simulink model "sla_vip_filter_vector"  (R2015b)
settings: Solver=FixedStepDiscrete  SolverMode=SingleTasking  StartTime=0.0  StopTime=1  RelTol=1e-3
PreLoadFcn:
  | Param_vip_vector
values from neighbouring files (symbols this model uses):
  Hvector = reshape(H, TAP*TAP, 1)    [Param_vip_vector.m]
  TAP = 5    [Param_vip_vector.m]
undefined symbols (not defined in the file or in its folder): LineBuf, TAPDly
libraries: simulink x11, dspobslib x10, visionsinks x3, dspsigattribs x2, dspvision x1, visionfilter x1, dspindex x1
settings Model: Creator=amatsumo  LastModifiedBy=amatsumo
settings DataIOCC: SaveFormat=Array  SignalLoggingSaveFormat=ModelDataLogs  SaveOutput=off  SignalLogging=off  SaveTime=off
settings OptimizationCC: BlockReduction=off  ConditionallyExecuteInputs=off  DefaultParameterBehavior=Inlined  ExpressionDepthLimit=2147483647
settings DebuggingCC: AlgebraicLoopMsg=error  UnderspecifiedInitializationDetection=Classic  MergeDetectMultiDrivingBlocksExec=none  SolverPrmCheckMsg=warning  InheritedTsInSrcMsg=none  SingleTaskRateTransMsg=error  ParameterPrecisionLossMsg=none  FcnCallInpInsideContextMsg=UseLocalSettings  StateNameClashWarn=warning
settings HardwareCC: ProdBitPerPointer=32  ProdLargestAtomicFloat=None  ProdIntDivRoundTo=Undefined  ProdEndianess=Unspecified  ProdWordSize=32  ProdHWDeviceType=ASIC/FPGA->ASIC/FPGA  TargetBitPerPointer=64  TargetLongLongMode=on  TargetIntDivRoundTo=Zero  TargetEndianess=LittleEndian  TargetWordSize=64  TargetHWDeviceType=MATLAB Host  ProdEqTarget=off
settings RTWCC: CustomInclude=C:\altera\12.0\modelsim_ase\include
settings GRTTargetCC: GeneratePreprocessorConditionals=Disable all  CombineOutputUpdateFcns=off  GRTInterface=on
settings ConfigComp: CovModelRefEnable=Off  CovSFcnEnable=off

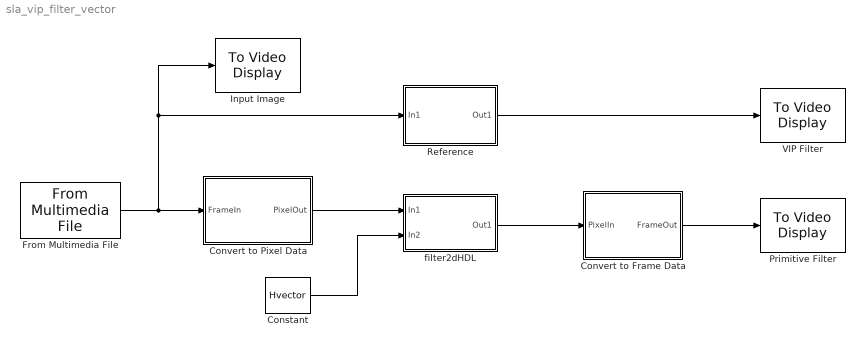
== system sla_vip_filter_vector ==
  Constant : Constant  Value=Hvector  OutDataTypeStr=dt_Hvector  SampleTime=-1
  Convert to Frame Data : Subsystem
  Convert to Pixel Data : Subsystem
  From Multimedia File : dspvision/From Multimedia File  inputFilename=vipmen.avi  loop=on  numPlays=inf  outputStreams=Video only  videoDataType=double  audioDataType=int16  inheritSampleTime=off  userDefinedSampleTime=1/24  noAudioOutput=off  isIntensityVideo=off  fourcc=Intensity  colorVideoFormat=Separate color signals  outputEOF=off  dataOrg=Column-major  audioFrameSize=1024  computeAudioFrameSize=off  outSamplingMode=Frame based
  Input Image : visionsinks/To Video Display  windowSizeMode=True size (1:1)  openAtMdlStart=on  fullScreen=off  videoWindowX=738  videoWindowY=-9  saveWindowSize=off  videoWindowWidth=160  videoWindowHeight=120  inputColorFormat=RGB  inputType=Obsolete  imagePorts=One multidimensional signal  OutputDevice=On-screen video monitor  dataOrg=Column-major  isWindowOpen=on
  Primitive Filter : visionsinks/To Video Display  windowSizeMode=True size (1:1)  openAtMdlStart=on  fullScreen=off  videoWindowX=1083  videoWindowY=-9  saveWindowSize=off  videoWindowWidth=160  videoWindowHeight=120  inputColorFormat=RGB  inputType=Obsolete  imagePorts=One multidimensional signal  OutputDevice=On-screen video monitor  dataOrg=Column-major  isWindowOpen=on
  Reference : Subsystem
  VIP Filter : visionsinks/To Video Display  windowSizeMode=True size (1:1)  openAtMdlStart=on  fullScreen=off  videoWindowX=908  videoWindowY=-9  saveWindowSize=off  videoWindowWidth=160  videoWindowHeight=120  inputColorFormat=RGB  inputType=Obsolete  imagePorts=One multidimensional signal  OutputDevice=On-screen video monitor  dataOrg=Column-major  isWindowOpen=on
  filter2dHDL : Subsystem
  wires:
  From Multimedia File/1 -> Convert to Pixel Data/1(FrameIn), Reference/1(In1), Input Image/1
  Reference/1(Out1) -> VIP Filter/1
  Convert to Frame Data/1(FrameOut) -> Primitive Filter/1
  Convert to Pixel Data/1(PixelOut) -> filter2dHDL/1(In1)
  filter2dHDL/1(Out1) -> Convert to Frame Data/1(PixelIn)
  Constant/1 -> filter2dHDL/2(In2)

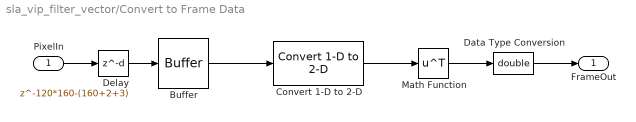
== system sla_vip_filter_vector/Convert to Frame Data ==
  PixelIn : Inport
  Buffer : Buffer  N=160*120  TreatMby1Signals=One channel
  Convert 1-D to 2-D : dspsigattribs/Convert 1-D to 2-D  M=160  N=120  frameBasedOut=off
  Data Type Conversion : DataTypeConversion  OutDataTypeStr=double  SaturateOnIntegerOverflow=on
  Delay : Delay  DelayLength=120*160-(160+2+3)  InitialCondition=0
  Math Function : Math  Operator=transpose  SaturateOnIntegerOverflow=on
  FrameOut : Outport
  wires:
  Buffer/1 -> Convert 1-D to 2-D/1
  Convert 1-D to 2-D/1 -> Math Function/1
  PixelIn/1 -> Delay/1
  Delay/1 -> Buffer/1
  Data Type Conversion/1 -> FrameOut/1
  Math Function/1 -> Data Type Conversion/1

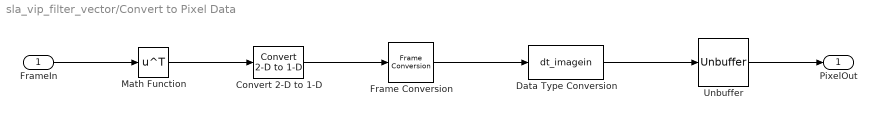
== system sla_vip_filter_vector/Convert to Pixel Data ==
  FrameIn : Inport
  Convert 2-D to 1-D : dspsigattribs/Convert 2-D to 1-D
  Data Type Conversion : DataTypeConversion  OutDataTypeStr=dt_imagein  SaturateOnIntegerOverflow=on
  Frame Conversion : FrameConversion  InheritSamplingMode=off
  Math Function : Math  Operator=transpose  SaturateOnIntegerOverflow=on
  Unbuffer : Unbuffer  SampleBasedProcessing=Same as frame based
  PixelOut : Outport
  wires:
  Frame Conversion/1 -> Data Type Conversion/1
  Convert 2-D to 1-D/1 -> Frame Conversion/1
  FrameIn/1 -> Math Function/1
  Unbuffer/1 -> PixelOut/1
  Data Type Conversion/1 -> Unbuffer/1
  Math Function/1 -> Convert 2-D to 1-D/1

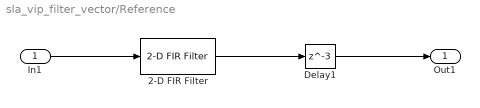
== system sla_vip_filter_vector/Reference ==
  In1 : Inport
  2-D FIR Filter : visionfilter/2-D FIR Filter  separable=off  filtSrc=Specify via dialog  filterMtrx=H  verticalFilter=[4 0]  horizontalFilter=[4 0]  outSize=Same as input port I  padType=Constant  padSrc=Specify via dialog  padVal=0  method=Convolution  firstCoeffMode=Binary point scaling  firstCoeffWordLength=8  firstCoeffFracLength=4  firstCoeffSignedness=Signed  firstCoeffDataTypeStr=fixdt(1,8,4)  firstCoeffLastDataTypeStr=fixdt(1,8,4)  firstCoeffMin=[]  firstCoeffMax=[]  outputMode=Binary point scaling  outputWordLength=20  outputFracLength=4  outputSignedness=Auto  outputDataTypeStr=fixdt([],20,4)  outputLastDataTypeStr=fixdt([],20,4)  outputMin=[]  outputMax=[]  accumDataTypeStr=Inherit: Same as product output  accumLastDataTypeStr=Inherit: Same as product output  prodOutputMode=Binary point scaling  prodOutputWordLength=16  prodOutputFracLength=4  prodOutputDataTypeStr=fixdt([],16,4)  prodOutputLastDataTypeStr=fixdt([],16,4)  roundingMode=Floor  overflowMode=on
  Delay1 : Delay  DelayLength=3  InitialCondition=0
  Out1 : Outport
  wires:
  Delay1/1 -> Out1/1
  2-D FIR Filter/1 -> Delay1/1
  In1/1 -> 2-D FIR Filter/1

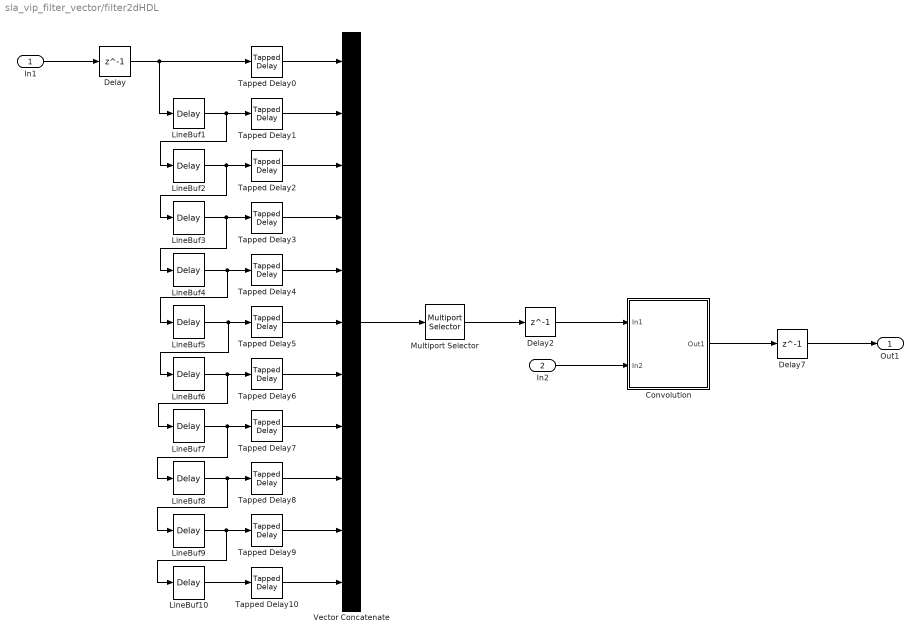
== system sla_vip_filter_vector/filter2dHDL ==
  In1 : Inport
  In2 : Inport  Port=2
  Convolution : Subsystem
  Delay : Delay  DelayLength=1
  Delay2 : Delay  DelayLength=1
  Delay7 : Delay  DelayLength=1
  LineBuf1 : dspobslib/Delay  InputProcessing=Columns as channels (frame based)  dly_unit=Samples  delay=LineBuf(1)  ic_detail=off  dif_ic_for_ch=off  dif_ic_for_dly=off  ic=0  reset_popup=None
  LineBuf10 : dspobslib/Delay  InputProcessing=Columns as channels (frame based)  dly_unit=Samples  delay=LineBuf(10)  ic_detail=off  dif_ic_for_ch=off  dif_ic_for_dly=off  ic=0  reset_popup=None
  LineBuf2 : dspobslib/Delay  InputProcessing=Columns as channels (frame based)  dly_unit=Samples  delay=LineBuf(2)  ic_detail=off  dif_ic_for_ch=off  dif_ic_for_dly=off  ic=0  reset_popup=None
  LineBuf3 : dspobslib/Delay  InputProcessing=Columns as channels (frame based)  dly_unit=Samples  delay=LineBuf(3)  ic_detail=off  dif_ic_for_ch=off  dif_ic_for_dly=off  ic=0  reset_popup=None
  LineBuf4 : dspobslib/Delay  InputProcessing=Columns as channels (frame based)  dly_unit=Samples  delay=LineBuf(4)  ic_detail=off  dif_ic_for_ch=off  dif_ic_for_dly=off  ic=0  reset_popup=None
  LineBuf5 : dspobslib/Delay  InputProcessing=Columns as channels (frame based)  dly_unit=Samples  delay=LineBuf(5)  ic_detail=off  dif_ic_for_ch=off  dif_ic_for_dly=off  ic=0  reset_popup=None
  LineBuf6 : dspobslib/Delay  InputProcessing=Columns as channels (frame based)  dly_unit=Samples  delay=LineBuf(6)  ic_detail=off  dif_ic_for_ch=off  dif_ic_for_dly=off  ic=0  reset_popup=None
  LineBuf7 : dspobslib/Delay  InputProcessing=Columns as channels (frame based)  dly_unit=Samples  delay=LineBuf(7)  ic_detail=off  dif_ic_for_ch=off  dif_ic_for_dly=off  ic=0  reset_popup=None
  LineBuf8 : dspobslib/Delay  InputProcessing=Columns as channels (frame based)  dly_unit=Samples  delay=LineBuf(8)  ic_detail=off  dif_ic_for_ch=off  dif_ic_for_dly=off  ic=0  reset_popup=None
  LineBuf9 : dspobslib/Delay  InputProcessing=Columns as channels (frame based)  dly_unit=Samples  delay=LineBuf(9)  ic_detail=off  dif_ic_for_ch=off  dif_ic_for_dly=off  ic=0  reset_popup=None
  Multiport Selector : dspindex/Multiport Selector  rowsOrCols=Rows  idxCellArray=[ 1: (TAP*TAP) ]  idxErrMode=Clip Index
  Tapped Delay0 : simulink/Discrete/Tapped Delay  vinit=0.0  samptime=-1  NumDelays=TAP  DelayOrder=Newest  includeCurrent=off
  Tapped Delay1 : simulink/Discrete/Tapped Delay  vinit=0.0  samptime=-1  NumDelays=TAPDly(1)  DelayOrder=Newest  includeCurrent=off
  Tapped Delay10 : simulink/Discrete/Tapped Delay  vinit=0.0  samptime=-1  NumDelays=TAPDly(10)  DelayOrder=Newest  includeCurrent=off
  Tapped Delay2 : simulink/Discrete/Tapped Delay  vinit=0.0  samptime=-1  NumDelays=TAPDly(2)  DelayOrder=Newest  includeCurrent=off
  Tapped Delay3 : simulink/Discrete/Tapped Delay  vinit=0.0  samptime=-1  NumDelays=TAPDly(3)  DelayOrder=Newest  includeCurrent=off
  Tapped Delay4 : simulink/Discrete/Tapped Delay  vinit=0.0  samptime=-1  NumDelays=TAPDly(4)  DelayOrder=Newest  includeCurrent=off
  Tapped Delay5 : simulink/Discrete/Tapped Delay  vinit=0.0  samptime=-1  NumDelays=TAPDly(5)  DelayOrder=Newest  includeCurrent=off
  Tapped Delay6 : simulink/Discrete/Tapped Delay  vinit=0.0  samptime=-1  NumDelays=TAPDly(6)  DelayOrder=Newest  includeCurrent=off
  Tapped Delay7 : simulink/Discrete/Tapped Delay  vinit=0.0  samptime=-1  NumDelays=TAPDly(7)  DelayOrder=Newest  includeCurrent=off
  Tapped Delay8 : simulink/Discrete/Tapped Delay  vinit=0.0  samptime=-1  NumDelays=TAPDly(8)  DelayOrder=Newest  includeCurrent=off
  Tapped Delay9 : simulink/Discrete/Tapped Delay  vinit=0.0  samptime=-1  NumDelays=TAPDly(9)  DelayOrder=Newest  includeCurrent=off
  Vector Concatenate : Concatenate  NumInputs=11
  Out1 : Outport
  wires:
  Delay7/1 -> Out1/1
  In1/1 -> Delay/1
  LineBuf1/1 -> LineBuf2/1, Tapped Delay1/1
  Delay/1 -> Tapped Delay0/1, LineBuf1/1
  Tapped Delay1/1 -> Vector Concatenate/2
  LineBuf2/1 -> Tapped Delay2/1, LineBuf3/1
  LineBuf3/1 -> LineBuf4/1, Tapped Delay3/1
  LineBuf4/1 -> LineBuf5/1, Tapped Delay4/1
  Tapped Delay2/1 -> Vector Concatenate/3
  Tapped Delay3/1 -> Vector Concatenate/4
  Tapped Delay4/1 -> Vector Concatenate/5
  Tapped Delay0/1 -> Vector Concatenate/1
  Tapped Delay5/1 -> Vector Concatenate/6
  LineBuf5/1 -> Tapped Delay5/1, LineBuf6/1
  Tapped Delay6/1 -> Vector Concatenate/7
  Vector Concatenate/1 -> Multiport Selector/1
  Tapped Delay7/1 -> Vector Concatenate/8
  LineBuf6/1 -> LineBuf7/1, Tapped Delay6/1
  LineBuf10/1 -> Tapped Delay10/1
  Tapped Delay8/1 -> Vector Concatenate/9
  Tapped Delay9/1 -> Vector Concatenate/10
  Tapped Delay10/1 -> Vector Concatenate/11
  LineBuf7/1 -> LineBuf8/1, Tapped Delay7/1
  LineBuf8/1 -> LineBuf9/1, Tapped Delay8/1
  LineBuf9/1 -> LineBuf10/1, Tapped Delay9/1
  Delay2/1 -> Convolution/1(In1)
  In2/1 -> Convolution/2(In2)
  Convolution/1(Out1) -> Delay7/1
  Multiport Selector/1 -> Delay2/1

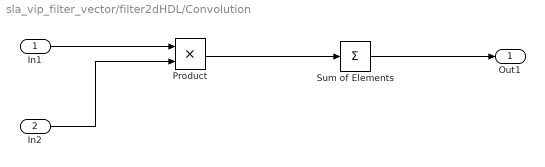
== system sla_vip_filter_vector/filter2dHDL/Convolution ==
  In1 : Inport
  In2 : Inport  Port=2
  Product : Product  OutDataTypeStr=dt_product  RndMeth=Zero
  Sum of Elements : Sum  Inputs=+  OutDataTypeStr=dt_sum  RndMeth=Nearest
  Out1 : Outport
  wires:
  Sum of Elements/1 -> Out1/1
  Product/1 -> Sum of Elements/1
  In2/1 -> Product/2
  In1/1 -> Product/1
